simulink model "AreaCoverageTestHarness"  (R2016b)
settings: Solver=FixedStepDiscrete  StartTime=0.0  StopTime=1000  FixedStep=0.0001  RelTol=1e-3  EnableMultiTasking=on
StopFcn:
  | if strcmp(get_param('AreaCoverageTestHarness/Robot/DetailedMap', 'Commented'), 'off')
  | evalin('base', 'MapCoveragePercent(roomSim)');
  | disp('STOP');
  | end
values from neighbouring files (symbols this model uses):
  BLOCK_SIZE = double(CAL_BLOCK_SIZE)    [AreaCoverageCalib.m]    (also in room_V1.m = 20; room_V2.m = 20; room_V3.m = 20)
  CAL_B_NmPerW = 1.5    [MotorConfigurationSheet.m]
  CAL_CurrentScaling_A = 0.04    [MotorConfigurationSheet.m]
  CAL_flux_e = 0.3    [MotorConfigurationSheet.m]
  CAL_flux_t = 3.0    (= 3)    [MotorConfigurationSheet.m]
  CAL_Inertia_J = 0.03    [MotorConfigurationSheet.m]
  CAL_Re_ohm = 0.5    [MotorConfigurationSheet.m]
  CAL_SimInduct_H = 0.001    [MotorConfigurationSheet.m]
  EAST = 0    [AreaCoverageCalib.m]
  ERRVAL = 5    [AreaCoverageCalib.m]
  gearRatio = 12    [AreaCoverageCalib.m]
  halfWheel_mm = 60    [AreaCoverageCalib.m]
  initXSim = 38    [AreaCoverageCalib.m]
  initYSim = 50    [AreaCoverageCalib.m]
  NORTH = 270    [AreaCoverageCalib.m]
  NVM_AngleStoreFlg = true    [AreaCoverageCalib.m]
  NVM_EAST = uint16(CAL_EAST)    [AreaCoverageCalib.m]
  NVM_NORTH = uint16(CAL_NORTH)    [AreaCoverageCalib.m]
  NVM_SOUTH = uint16(CAL_SOUTH)    [AreaCoverageCalib.m]
  NVM_WEST = uint16(CAL_WEST)    [AreaCoverageCalib.m]
  ROB_LENG_m = 0.25    [AreaCoverageCalib.m]
  ROBO_LENG = 30    [realMapPlotter.m]    (also in roomDrawing.m)
  ROOM_SIDE_SIZE = double(CAL_ROOM_SIDE_SIZE)    [AreaCoverageCalib.m]    (also in room_V1.m = 20; room_V2.m = 20; room_V3.m = 20)
  SAMPLE_TIME = 0.001    [AreaCoverageCalib.m]
  SOUTH = 90    [AreaCoverageCalib.m]
  thetaMapBp = [0 : 0.1 : 360]    [AreaCoverageCalib.m]
  thetaMapTb = [thetaMapTb1, thetaMapTb2, thetaMapTb3, thetaMapTb4, thetaMapTb5]    [AreaCoverageCalib.m]
  WEST = 180    [AreaCoverageCalib.m]
undefined symbols (not defined in the file or in its folder): CAL_WheelDiameter_cm, DiscIntNeverNeededParam, ENU_BACKWARD, ENU_FORWARD
libraries: simulink x3, RobotControlLib x1
(part 1 of 3)
settings Model: Creator=oelkawok  LastModifiedBy=oelkawok
settings OptimizationCC: DefaultParameterBehavior=Inlined  UseDivisionForNetSlopeComputation=on  DefaultUnderspecifiedDataType=single  EfficientFloat2IntCast=on  LifeSpan=Inf
settings DebuggingCC: ConsistencyChecking=warning  SignalInfNanChecking=error  SignalRangeChecking=error  ReadBeforeWriteMsg=EnableAllAsError  WriteAfterWriteMsg=EnableAllAsError  WriteAfterReadMsg=EnableAllAsError  AlgebraicLoopMsg=error  ArtificialAlgebraicLoopMsg=error  SaveWithParameterizedLinksMsg=error  SignalResolutionControl=TryResolveAllWithWarning  BlockPriorityViolationMsg=error  MinStepSizeMsg=error  SolverPrmCheckMsg=error  InheritedTsInSrcMsg=error  SingleTaskRateTransMsg=error  TasksWithSamePriorityMsg=error  SigSpecEnsureSampleTimeMsg=error  CheckMatrixSingularityMsg=error  IntegerOverflowMsg=error  ParameterUnderflowMsg=error  UnderSpecifiedDataTypeMsg=warning  UnnecessaryDatatypeConvMsg=warning  VectorMatrixConversionMsg=error  SignalLabelMismatchMsg=error  UnconnectedLineMsg=error  SFcnCompatibilityMsg=warning  UniqueDataStoreMsg=error  BusObjectLabelMismatch=error  RootOutportRequireBusObject=error  AssertControl=DisableAll  ModelReferenceIOMsg=error  ModelReferenceVersionMismatchMessage=error  ModelReferenceIOMismatchMessage=error  UnknownTsInhSupMsg=error  ModelReferenceDataLoggingMessage=error  StateNameClashWarn=warning  StrictBusMsg=ErrorOnBusTreatedAsVector  NonBusSignalsTreatedAsBus=error  SFUnusedDataAndEventsDiag=error  SFInvalidInputDataAccessInChartInitDiag=error  SFTransitionOutsideNaturalParentDiag=error  SFUnreachableExecutionPathDiag=error  SFUndirectedBroadcastEventsDiag=error  SFTransitionActionBeforeConditionDiag=error  SFTemporalDelaySmallerThanSampleTimeDiag=error  SFSelfTransitionDiag=error  SFExecutionAtInitializationDiag=none  SFMachineParentedDataDiag=error
settings HardwareCC: ProdLongLongMode=on
settings RTWCC: SystemTargetFile=ert.tlc  TemplateMakefile=ert_default_tmf  Description=Embedded Coder  GenerateReport=on  IncludeHyperlinkInReport=on  LaunchReport=on  GenerateTraceInfo=on  GenerateTraceReport=on  GenerateTraceReportSl=on  GenerateTraceReportSf=on  GenerateTraceReportEml=on
settings CodeAppCC: ForceParamTrailComments=on  IgnoreCustomStorageClasses=off  OperatorAnnotations=on  SimulinkDataObjDesc=on  SFDataObjDesc=on  MATLABFcnDesc=on  InsertBlockDesc=on  MATLABSourceComments=on  ReqsInCode=on
settings ERTTargetCC: GenerateSampleERTMain=on  InlinedParameterPlacement=NonHierarchical  ERTCustomFileTemplate=example_file_process.tlc
settings ConfigComp: CovScope=ReferencedModels  CovIncludeTopModel=off  CovMetricSettings=dw  CovHtmlReporting=on  CovSaveCumulativeToWorkspaceVar=on  CovSaveSingleToWorkspaceVar=on  CovExternalEMLEnable=off

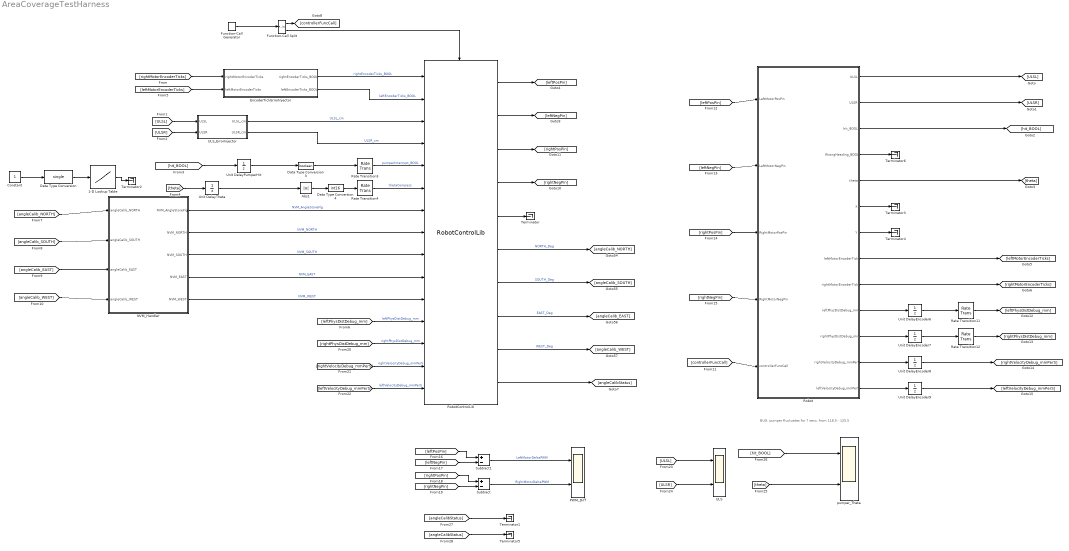
== system AreaCoverageTestHarness ==
  note: BUG: pumper fluctuates for 7 secs. from 118.5 - 125.5
  1-D Lookup Table : Lookup_n-D  NumberOfTableDimensions=1  BreakpointsForDimension1=thetaMapBp  Table=thetaMapTb  ExtrapMethod=Clip  InternalRulePriority=Speed  RndMeth=Simplest  InputSameDT=on
  Abs1 : Abs
  Constant : Constant
  Data Type Conversion : DataTypeConversion  OutDataTypeStr=single
  Data Type Conversion3 : DataTypeConversion  OutDataTypeStr=boolean
  Data Type Conversion4 : DataTypeConversion  OutDataTypeStr=int16
  EncoderTickErrorInjector : Subsystem
  Function-Call Generator : simulink/Ports & Subsystems/Function-Call Generator  sample_time=0.001  numberOfIterations=1
  Function-Call Split : FunctionCallSplit  IconShape=distinctive  NumOutputPorts=2  OutputPortLayout=default
  NVM_Handler : Subsystem
  PWM_Diff : Scope  NumInputPorts=2
  Rate Transition{3..4,11..12} (4 alike) : RateTransition
  Robot : Subsystem
  RobotControlLib : RobotControlLib/RobotControlLib  Description=Main Control Function
  Subtract : Sum  Inputs=+-  OutDataTypeStr=int16
  Subtract1 : Sum  Inputs=+-  OutDataTypeStr=int16
  Terminator{,1..6} (7 alike) : Terminator
  ULS : Scope  NumInputPorts=2
  ULS_ErrorInjector : Subsystem
  Unit DelayEncoder{6..9} (4 alike) : UnitDelay  SampleTime=-1
  Unit DelayPumperHit : UnitDelay  SampleTime=-1
      settings: AttributesFormatString=Init: %<InitialCondition>
  Unit DelayTheta : UnitDelay  InitialCondition=NORTH  SampleTime=-1
      settings: AttributesFormatString=%<InitialCondition>
  pumper_Theta : Scope  NumInputPorts=2
  wires:
  Data Type Conversion3/1 -> Rate Transition3/1
  Unit DelayPumperHit/1 -> Data Type Conversion3/1
  Abs1/1 -> Data Type Conversion4/1
  Robot/9(rightMotorEncoderTicks) -> [rightMotorEncoderTicks]
  Robot/1(ULSL) -> [ULSL]
  Robot/2(ULSR) -> [ULSR]
  Robot/3(hit_BOOL) -> [hit_BOOL]
  Robot/5(theta) -> [theta]
  Robot/8(leftMotorEncoderTicks) -> [leftMotorEncoderTicks]
  [hit_BOOL] -> Unit DelayPumperHit/1
  [theta] -> Unit DelayTheta/1
  RobotControlLib/10 -> [angleCalibStatus]
  RobotControlLib/6 -> [angleCalib_NORTH]  "NORTH_Deg"
  RobotControlLib/7 -> [angleCalib_SOUTH]  "SOUTH_Deg"
  RobotControlLib/8 -> [angleCalib_EAST]  "EAST_Deg"
  RobotControlLib/9 -> [angleCalib_WEST]  "WEST_Deg"
  Function-Call Generator/1 -> Function-Call Split/1
  [controllerFuncCall] -> Robot/5(controllerFuncCall)
  Function-Call Split/1 -> [controllerFuncCall]
  Function-Call Split/2 -> RobotControlLib/Trigger
  Rate Transition3/1 -> RobotControlLib/5  "pumperInterrupt_BOOL"
  Rate Transition4/1 -> RobotControlLib/6  "thetaCompass"
  Robot/10(leftPhysDistDebug_mm) -> Unit DelayEncoder6/1
  Robot/11(rightPhysDistDebug_mm) -> Unit DelayEncoder7/1
  Robot/12(rightVelocityDebug_mmPerS) -> Unit DelayEncoder8/1
  Robot/13(leftVelocityDebug_mmPerS) -> Unit DelayEncoder9/1
  Subtract/1 -> PWM_Diff/2  "RightMotorDeltaPWM"
  Subtract1/1 -> PWM_Diff/1  "LeftMotorDeltaPWM"
  RobotControlLib/1 -> [leftPosPin]
  RobotControlLib/2 -> [leftNegPin]
  RobotControlLib/3 -> [rightPosPin]
  RobotControlLib/4 -> [rightNegPin]
  [leftPosPin] -> Robot/1(LeftMotorPosPin)
  [leftNegPin] -> Robot/2(LeftMotorNegPin)
  [rightPosPin] -> Robot/3(RightMotorPosPin)
  [rightNegPin] -> Robot/4(RightMotorNegPin)
  [leftNegPin] -> Subtract1/2
  [leftPosPin] -> Subtract1/1
  [rightNegPin] -> Subtract/2
  [rightPosPin] -> Subtract/1
  [angleCalib_SOUTH] -> NVM_Handler/2(angleCalib_SOUTH)
  [angleCalib_NORTH] -> NVM_Handler/1(angleCalib_NORTH)
  [angleCalib_EAST] -> NVM_Handler/3(angleCalib_EAST)
  [angleCalib_WEST] -> NVM_Handler/4(angleCalib_WEST)
  Unit DelayEncoder6/1 -> Rate Transition11/1
  Rate Transition11/1 -> [leftPhysDistDebug_mm]
  [leftPhysDistDebug_mm] -> RobotControlLib/12  "leftPhysDistDebug_mm"
  Unit DelayEncoder7/1 -> Rate Transition12/1
  Rate Transition12/1 -> [rightPhysDistDebug_mm]
  [rightPhysDistDebug_mm] -> RobotControlLib/13  "rightPhysDistDebug_mm"
  Unit DelayEncoder8/1 -> [rightVelocityDebug_mmPerS]
  [rightVelocityDebug_mmPerS] -> RobotControlLib/14  "rightVelocityDebug_mmPerS"
  Unit DelayEncoder9/1 -> [leftVelocityDebug_mmPerS]
  [leftVelocityDebug_mmPerS] -> RobotControlLib/15  "leftVelocityDebug_mmPerS"
  NVM_Handler/5(NVM_WEST) -> RobotControlLib/11  "NVM_WEST"
  NVM_Handler/4(NVM_EAST) -> RobotControlLib/10  "NVM_EAST"
  NVM_Handler/3(NVM_SOUTH) -> RobotControlLib/9  "NVM_SOUTH"
  NVM_Handler/2(NVM_NORTH) -> RobotControlLib/8  "NVM_NORTH"
  NVM_Handler/1(NVM_AngleStoreFlg) -> RobotControlLib/7  "NVM_AngleStoreFlg"
  ULS_ErrorInjector/1(ULSL_cm) -> RobotControlLib/3  "ULSL_cm"
  ULS_ErrorInjector/2(ULSR_cm) -> RobotControlLib/4  "ULSR_cm"
  [ULSL] -> ULS_ErrorInjector/1(ULSL)
  [ULSR] -> ULS_ErrorInjector/2(ULSR)
  EncoderTickErrorInjector/1(rightEncoderTicks_BOOL) -> RobotControlLib/1  "rightEncoderTicks_BOOL"
  EncoderTickErrorInjector/2(leftEncoderTicks_BOOL) -> RobotControlLib/2  "leftEncoderTicks_BOOL"
  [leftMotorEncoderTicks] -> EncoderTickErrorInjector/2(leftMotorEncoderTicks)
  [rightMotorEncoderTicks] -> EncoderTickErrorInjector/1(rightMotorEncoderTicks)
  [ULSL] -> ULS/1
  [ULSR] -> ULS/2
  [theta] -> pumper_Theta/2
  [hit_BOOL] -> pumper_Theta/1
  Data Type Conversion4/1 -> Rate Transition4/1
  Unit DelayTheta/1 -> Abs1/1
  RobotControlLib/5 -> Terminator/1
  [angleCalibStatus] -> Terminator1/1
  Constant/1 -> Data Type Conversion/1
  1-D Lookup Table/1 -> Terminator2/1
  Robot/6(X) -> Terminator3/1
  Robot/7(Y) -> Terminator4/1
  [angleCalibStatus] -> Terminator5/1
  Robot/4(WrongHeading_BOOL) -> Terminator6/1
  Data Type Conversion/1 -> 1-D Lookup Table/1

== system AreaCoverageTestHarness/EncoderTickErrorInjector ==
  rightMotorEncoderTicks : Inport
  leftMotorEncoderTicks : Inport  Port=2
  Constant4 : Constant  Value=false
  Constant5 : Constant  Value=false
  Data Type Conversion1 : DataTypeConversion  OutDataTypeStr=boolean
  Data Type Conversion2 : DataTypeConversion  OutDataTypeStr=boolean
  Manual Switch2 : ManualSwitch
  Manual Switch3 : ManualSwitch
  Rate Transition : RateTransition
  Rate Transition5 : RateTransition
  Unit DelayEncoder : UnitDelay  SampleTime=-1
      settings: AttributesFormatString=init: %<InitialCondition>
  Unit DelayEncoder1 : UnitDelay  SampleTime=-1
      settings: AttributesFormatString=init: %<InitialCondition>
  rightEncoderTicks_BOOL : Outport
  leftEncoderTicks_BOOL : Outport  Port=2
  wires:
  Data Type Conversion2/1 -> Manual Switch3/1
  Unit DelayEncoder/1 -> Data Type Conversion2/1
  Constant5/1 -> Manual Switch3/2
  Manual Switch3/1 -> Rate Transition/1
  Rate Transition/1 -> rightEncoderTicks_BOOL/1
  Unit DelayEncoder1/1 -> Data Type Conversion1/1
  Constant4/1 -> Manual Switch2/2
  Manual Switch2/1 -> Rate Transition5/1
  Rate Transition5/1 -> leftEncoderTicks_BOOL/1
  Data Type Conversion1/1 -> Manual Switch2/1
  rightMotorEncoderTicks/1 -> Unit DelayEncoder/1
  leftMotorEncoderTicks/1 -> Unit DelayEncoder1/1

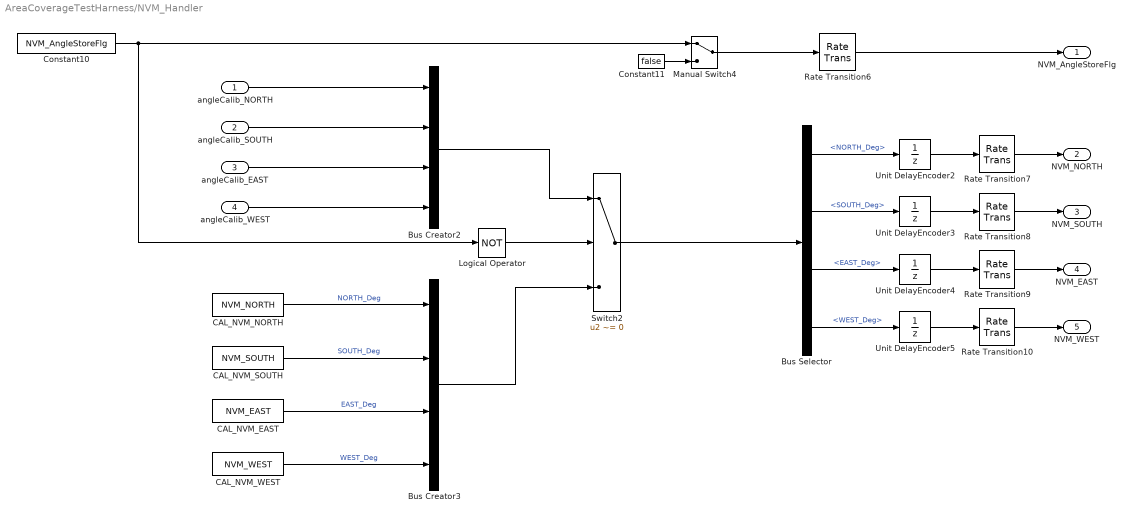
== system AreaCoverageTestHarness/NVM_Handler ==
  angleCalib_NORTH : Inport
  angleCalib_SOUTH : Inport  Port=2
  angleCalib_EAST : Inport  Port=3
  angleCalib_WEST : Inport  Port=4
  Bus Creator2 : BusCreator  Inputs=4
  Bus Creator3 : BusCreator  Inputs=4
  Bus Selector : BusSelector  OutputSignals=NORTH_Deg,SOUTH_Deg,EAST_Deg,WEST_Deg
  CAL_NVM_EAST : Constant  Value=NVM_EAST
  CAL_NVM_NORTH : Constant  Value=NVM_NORTH
  CAL_NVM_SOUTH : Constant  Value=NVM_SOUTH
  CAL_NVM_WEST : Constant  Value=NVM_WEST
  Constant10 : Constant  Value=NVM_AngleStoreFlg
  Constant11 : Constant  Value=false
  Logical Operator : Logic  Operator=NOT  IconShape=distinctive  AllPortsSameDT=off  OutDataTypeStr=boolean
  Manual Switch4 : ManualSwitch
  Rate Transition{6..10} (5 alike) : RateTransition
  Switch2 : Switch  Criteria=u2 ~= 0
  Unit DelayEncoder{2..5} (4 alike) : UnitDelay  SampleTime=-1
  NVM_AngleStoreFlg : Outport
  NVM_NORTH : Outport  Port=2
  NVM_SOUTH : Outport  Port=3
  NVM_EAST : Outport  Port=4
  NVM_WEST : Outport  Port=5
  wires:
  Constant10/1 -> Logical Operator/1, Manual Switch4/1
  Bus Creator2/1 -> Switch2/1
  Bus Creator3/1 -> Switch2/3
  Bus Selector/3 -> Unit DelayEncoder4/1  "<EAST_Deg>"
  Switch2/1 -> Bus Selector/1
  Bus Selector/4 -> Unit DelayEncoder5/1  "<WEST_Deg>"
  CAL_NVM_NORTH/1 -> Bus Creator3/1  "NORTH_Deg"
  CAL_NVM_EAST/1 -> Bus Creator3/3  "EAST_Deg"
  CAL_NVM_WEST/1 -> Bus Creator3/4  "WEST_Deg"
  Bus Selector/1 -> Unit DelayEncoder2/1  "<NORTH_Deg>"
  CAL_NVM_SOUTH/1 -> Bus Creator3/2  "SOUTH_Deg"
  Bus Selector/2 -> Unit DelayEncoder3/1  "<SOUTH_Deg>"
  Logical Operator/1 -> Switch2/2
  angleCalib_NORTH/1 -> Bus Creator2/1
  angleCalib_SOUTH/1 -> Bus Creator2/2
  angleCalib_WEST/1 -> Bus Creator2/4
  angleCalib_EAST/1 -> Bus Creator2/3
  Rate Transition10/1 -> NVM_WEST/1
  Rate Transition7/1 -> NVM_NORTH/1
  Rate Transition8/1 -> NVM_SOUTH/1
  Rate Transition9/1 -> NVM_EAST/1
  Manual Switch4/1 -> Rate Transition6/1
  Constant11/1 -> Manual Switch4/2
  Rate Transition6/1 -> NVM_AngleStoreFlg/1
  Unit DelayEncoder2/1 -> Rate Transition7/1
  Unit DelayEncoder3/1 -> Rate Transition8/1
  Unit DelayEncoder4/1 -> Rate Transition9/1
  Unit DelayEncoder5/1 -> Rate Transition10/1

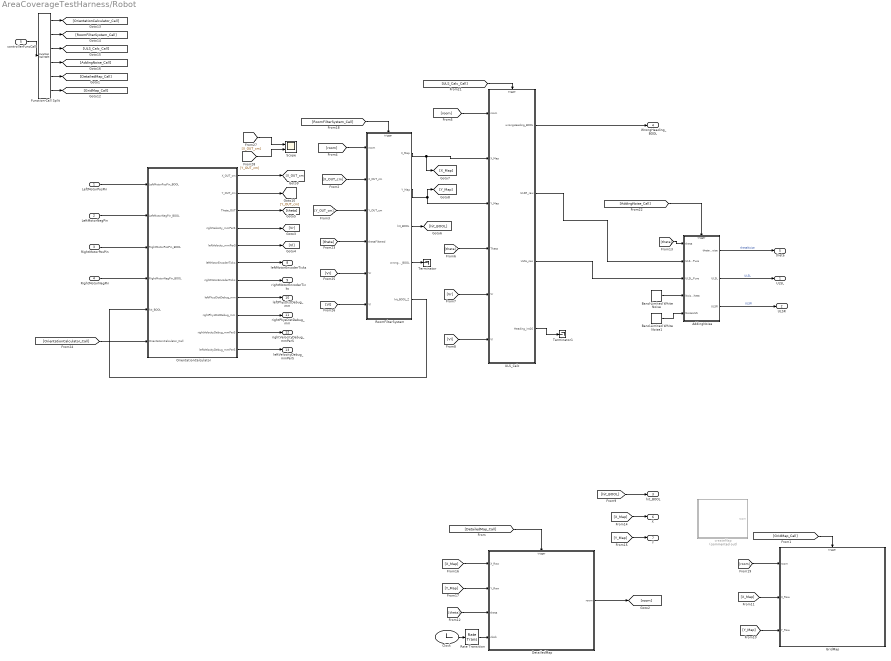
== system AreaCoverageTestHarness/Robot ==
  LeftMotorPosPin : Inport
  LeftMotorNegPin : Inport  Port=2
  RightMotorPosPin : Inport  Port=3
  RightMotorNegPin : Inport  Port=4
  controllerFuncCall : Inport  Port=5
  AddingNoise : Subsystem
  Band-Limited White Noise : simulink/Sources/Band-Limited White Noise  Cov=[0.001]  Ts=0.001  seed=[23]
  Band-Limited White Noise1 : simulink/Sources/Band-Limited White Noise  Cov=[0.001]  Ts=0.001  seed=[23]
  Clock : Clock
      settings: Decimation=100
  DetailedMap : Subsystem
  Function-Call Split : FunctionCallSplit  IconShape=distinctive  NumOutputPorts=6  OutputPortLayout=default
  GridMap : Subsystem
  OrientationCalculator : Subsystem
  Rate Transition : RateTransition
  RoomFilterSystem : Subsystem
  Scope : Scope  NumInputPorts=2
  Terminator : Terminator
  Terminator1 : Terminator
  ULS_Calc : Subsystem
  createMap : Subsystem  Commented=on
  ULSL : Outport
  ULSR : Outport  Port=2
  hit_BOOL : Outport  Port=3
  WrongHeading_BOOL : Outport  Port=4
  theta : Outport  Port=5
  X : Outport  Port=6
  Y : Outport  Port=7
  leftMotorEncoderTicks : Outport  Port=8
  rightMotorEncoderTicks : Outport  Port=9
  leftPhysDistDebug_mm : Outport  Port=10
  rightPhysDistDebug_mm : Outport  Port=11
  rightVelocityDebug_mmPerS : Outport  Port=12
  leftVelocityDebug_mmPerS : Outport  Port=13
  wires:
  RightMotorNegPin/1 -> OrientationCalculator/4(RightMotorNegPin_BOOL)
  RightMotorPosPin/1 -> OrientationCalculator/3(RightMotorPosPin_BOOL)
  OrientationCalculator/3(Theta_OUT) -> [theta]
  OrientationCalculator/4(rightVelocity_mmPerS) -> [Vr]
  RoomFilterSystem/3(hit_BOOL) -> [hit_BOOL]
  RoomFilterSystem/5(hit_BOOL_Z) -> OrientationCalculator/5(hit_BOOL)
  [room] -> RoomFilterSystem/1(room)
  [room] -> ULS_Calc/1(room)
  [theta] -> ULS_Calc/4(Theta)
  [Vr] -> ULS_Calc/5(Vr)
  [Vl] -> ULS_Calc/6(Vl)
  [hit_BOOL] -> hit_BOOL/1
  ULS_Calc/1(wrongHeading_BOOL) -> WrongHeading_BOOL/1
  RoomFilterSystem/2(Y_Map) -> ULS_Calc/3(Y_Map), [Y_Map]
  RoomFilterSystem/1(X_Map) -> [X_Map], ULS_Calc/2(X_Map)
  [Y_Map] -> Y/1
  [X_Map] -> X/1
  OrientationCalculator/1(X_OUT_cm) -> [X_OUT_cm]
  OrientationCalculator/2(Y_OUT_cm) -> [Y_OUT_cm]
  [X_Map] -> DetailedMap/1(X_Raw)
  [Y_Map] -> DetailedMap/2(Y_Raw)
  [theta] -> DetailedMap/3(theta)
  [X_Map] -> GridMap/2(X_Raw)
  [Y_Map] -> GridMap/3(Y_Raw)
  [room] -> GridMap/1(room)
  DetailedMap/1(room) -> [room]
  AddingNoise/2(ULSL) -> ULSL/1  "ULSL"
  AddingNoise/3(ULSR) -> ULSR/1  "ULSR"
  OrientationCalculator/6(leftMotorEncoderTicks) -> leftMotorEncoderTicks/1
  OrientationCalculator/7(rightMotorEncoderTicks) -> rightMotorEncoderTicks/1
  RoomFilterSystem/4(wrongHeading_BOOL) -> Terminator/1
  AddingNoise/1(thetaNoise) -> theta/1  "thetaNoise"
  [theta] -> AddingNoise/1(theta)
  ULS_Calc/3(ULSL_raw) -> AddingNoise/3(ULSL_Pure)
  [RoomFilterSystem_Call] -> RoomFilterSystem/Trigger
  [ULS_Calc_Call] -> ULS_Calc/Trigger
  [OrientationCalculator_Call] -> OrientationCalculator/6(OrientationCalculator_Call)
  controllerFuncCall/1 -> Function-Call Split/1
  ULS_Calc/2(ULSR_raw) -> AddingNoise/2(ULSR_Pure)
  [AddingNoise_Call] -> AddingNoise/Trigger
  Function-Call Split/4 -> [AddingNoise_Call]
  Function-Call Split/3 -> [ULS_Calc_Call]
  Function-Call Split/2 -> [RoomFilterSystem_Call]
  Function-Call Split/1 -> [OrientationCalculator_Call]
  Band-Limited White Noise1/1 -> AddingNoise/5(NoiseULS)
  Band-Limited White Noise/1 -> AddingNoise/4(NoiseTheta)
  OrientationCalculator/8(leftPhysDistDebug_mm) -> leftPhysDistDebug_mm/1
  OrientationCalculator/9(rightPhysDistDebug_mm) -> rightPhysDistDebug_mm/1
  OrientationCalculator/11(leftVelocityDebug_mmPerS) -> leftVelocityDebug_mmPerS/1
  OrientationCalculator/10(rightVelocityDebug_mmPerS) -> rightVelocityDebug_mmPerS/1
  LeftMotorPosPin/1 -> OrientationCalculator/1(LeftMotorPosPin_BOOL)
  LeftMotorNegPin/1 -> OrientationCalculator/2(LeftMotorNegPin_BOOL)
  Function-Call Split/5 -> [DetailedMap_Call]
  Function-Call Split/6 -> [GridMap_Call]
  [DetailedMap_Call] -> DetailedMap/Trigger
  [GridMap_Call] -> GridMap/Trigger
  Clock/1 -> Rate Transition/1
  Rate Transition/1 -> DetailedMap/4(clock)
  [X_OUT_cm] -> RoomFilterSystem/2(X_OUT_cm)
  [Y_OUT_cm] -> RoomFilterSystem/3(Y_OUT_cm)
  [theta] -> RoomFilterSystem/4(thetaFiltered)
  [Vr] -> RoomFilterSystem/5(Vr)
  OrientationCalculator/5(leftVelocity_mmPerS) -> [Vl]
  [Vl] -> RoomFilterSystem/6(Vl)
  [X_OUT_cm] -> Scope/1
  [Y_OUT_cm] -> Scope/2
  ULS_Calc/4(Heading_int16) -> Terminator1/1

== system AreaCoverageTestHarness/ULS_ErrorInjector ==
  ULSL : Inport
  ULSR : Inport  Port=2
  Abs2 : Abs
  Abs3 : Abs
  Constant : Constant  Value=0  OutDataTypeStr=uint16
  Constant2 : Constant  Value=0  OutDataTypeStr=uint16
  Data Type Conversion : DataTypeConversion  OutDataTypeStr=uint16
  Data Type Conversion1 : DataTypeConversion  OutDataTypeStr=uint16
  Manual Switch : ManualSwitch
  Manual Switch1 : ManualSwitch
  Rate Transition1 : RateTransition
  Rate Transition2 : RateTransition
  Unit DelayULSL : UnitDelay  InitialCondition=1  SampleTime=-1
  Unit DelayULSR : UnitDelay  InitialCondition=1  SampleTime=-1
  ULSL_cm : Outport
  ULSR_cm : Outport  Port=2
  wires:
  Manual Switch/1 -> Rate Transition1/1
  Abs3/1 -> Data Type Conversion1/1
  Abs2/1 -> Data Type Conversion/1
  Unit DelayULSL/1 -> Abs3/1
  Data Type Conversion/1 -> Manual Switch/1
  Data Type Conversion1/1 -> Manual Switch1/1
  Constant/1 -> Manual Switch/2
  Constant2/1 -> Manual Switch1/2
  Manual Switch1/1 -> Rate Transition2/1
  Unit DelayULSR/1 -> Abs2/1
  Rate Transition1/1 -> ULSL_cm/1
  Rate Transition2/1 -> ULSR_cm/1
  ULSR/1 -> Unit DelayULSL/1
  ULSL/1 -> Unit DelayULSR/1

== system AreaCoverageTestHarness/Robot/AddingNoise ==
  theta : Inport
  ULSR_Pure : Inport  Port=2
  ULSL_Pure : Inport  Port=3
  NoiseTheta : Inport  Port=4
  NoiseULS : Inport  Port=5
  function : TriggerPort  TriggerType=function-call  VariantControl=Variant
  Sum : Sum  Inputs=|++
  Sum1 : Sum  Inputs=|++
  Sum2 : Sum  Inputs=++|
  thetaNoise : Outport
  ULSL : Outport  Port=2
      settings: AttributesFormatString=%<OutputWhenDisabled>
  ULSR : Outport  Port=3
      settings: AttributesFormatString=%<OutputWhenDisabled>
  wires:
  NoiseTheta/1 -> Sum/2
  Sum/1 -> thetaNoise/1
  theta/1 -> Sum/1  "theta"
  ULSR_Pure/1 -> Sum1/1
  ULSL_Pure/1 -> Sum2/2
  NoiseULS/1 -> Sum1/2, Sum2/1
  Sum1/1 -> ULSR/1
  Sum2/1 -> ULSL/1

== system AreaCoverageTestHarness/Robot/DetailedMap ==
  X_Raw : Inport
  Y_Raw : Inport  Port=2
  theta : Inport  Port=3
  clock : Inport  Port=4
  function : TriggerPort  TriggerType=function-call  VariantControl=Variant
  MATLAB Function : MATLAB Function  TreatAsAtomicUnit=on
  createMap : Subsystem  Variant=on  OverrideUsingVariant=Variant
  room : Outport
  wires:
  theta/1 -> MATLAB Function/4(Theta)
  createMap/1(room) -> room/1, MATLAB Function/1(room)
  X_Raw/1 -> MATLAB Function/2(X)
  Y_Raw/1 -> MATLAB Function/3(Y)
  clock/1 -> MATLAB Function/5(clock)

== system AreaCoverageTestHarness/Robot/GridMap ==
  room : Inport
  X_Raw : Inport  Port=2
  Y_Raw : Inport  Port=3
  function : TriggerPort  TriggerType=function-call  VariantControl=Variant
  MATLAB Function : MATLAB Function  TreatAsAtomicUnit=on
  wires:
  Y_Raw/1 -> MATLAB Function/3(Y)
  X_Raw/1 -> MATLAB Function/2(X)
  room/1 -> MATLAB Function/1(room)

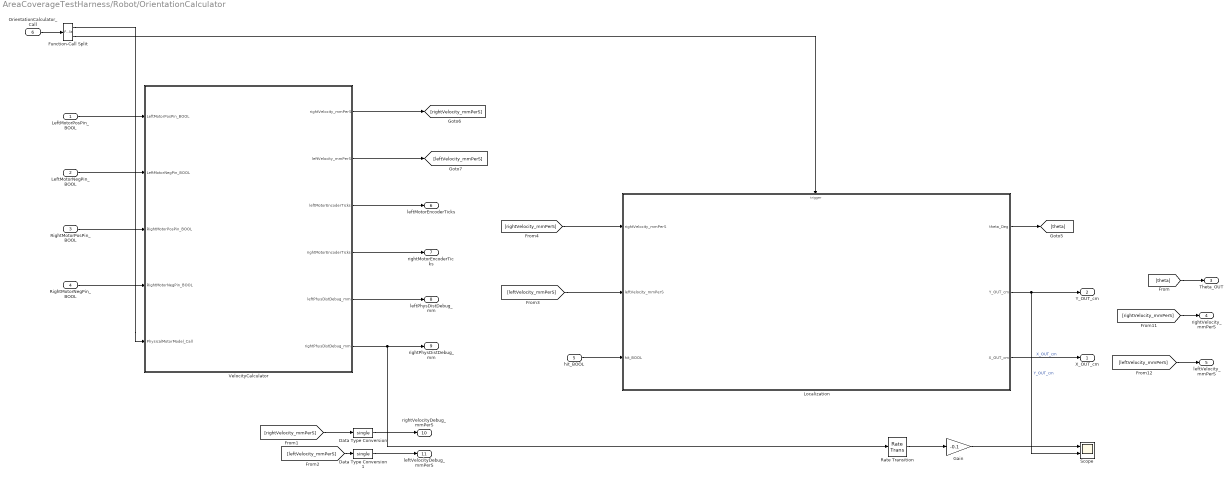
== system AreaCoverageTestHarness/Robot/OrientationCalculator ==
  LeftMotorPosPin_BOOL : Inport
  LeftMotorNegPin_BOOL : Inport  Port=2
  RightMotorPosPin_BOOL : Inport  Port=3
  RightMotorNegPin_BOOL : Inport  Port=4
  hit_BOOL : Inport  Port=5
  OrientationCalculator_Call : Inport  Port=6
  Data Type Conversion : DataTypeConversion  OutDataTypeStr=single
  Data Type Conversion1 : DataTypeConversion  OutDataTypeStr=single
  Function-Call Split : FunctionCallSplit  IconShape=distinctive  NumOutputPorts=2
  Gain : Gain  Gain=-0.1
  Localization : Subsystem
  Rate Transition : RateTransition
  Scope : Scope  NumInputPorts=2
  VelocityCalculator : Subsystem
  X_OUT_cm : Outport
  Y_OUT_cm : Outport  Port=2
  Theta_OUT : Outport  Port=3
  rightVelocity_mmPerS : Outport  Port=4
  leftVelocity_mmPerS : Outport  Port=5
  leftMotorEncoderTicks : Outport  Port=6
  rightMotorEncoderTicks : Outport  Port=7
  leftPhysDistDebug_mm : Outport  Port=8
  rightPhysDistDebug_mm : Outport  Port=9
  rightVelocityDebug_mmPerS : Outport  Port=10
  leftVelocityDebug_mmPerS : Outport  Port=11
  wires:
  [leftVelocity_mmPerS] -> leftVelocity_mmPerS/1
  [rightVelocity_mmPerS] -> rightVelocity_mmPerS/1
  Localization/1(theta_Deg) -> [theta]
  [theta] -> Theta_OUT/1
  VelocityCalculator/3(leftMotorEncoderTicks) -> leftMotorEncoderTicks/1
  VelocityCalculator/4(rightMotorEncoderTicks) -> rightMotorEncoderTicks/1
  Localization/2(Y_OUT_cm) -> Scope/2, Y_OUT_cm/1  "Y_OUT_cm"
  Localization/3(X_OUT_cm) -> X_OUT_cm/1  "X_OUT_cm"
  hit_BOOL/1 -> Localization/3(hit_BOOL)
  LeftMotorPosPin_BOOL/1 -> VelocityCalculator/1(LeftMotorPosPin_BOOL)
  RightMotorNegPin_BOOL/1 -> VelocityCalculator/4(RightMotorNegPin_BOOL)
  RightMotorPosPin_BOOL/1 -> VelocityCalculator/3(RightMotorPosPin_BOOL)
  LeftMotorNegPin_BOOL/1 -> VelocityCalculator/2(LeftMotorNegPin_BOOL)
  VelocityCalculator/1(rightVelocity_mmPerS) -> [rightVelocity_mmPerS]
  VelocityCalculator/2(leftVelocity_mmPerS) -> [leftVelocity_mmPerS]
  OrientationCalculator_Call/1 -> Function-Call Split/1
  Function-Call Split/2 -> Localization/Trigger
  Function-Call Split/1 -> VelocityCalculator/5(PhysicalMotorModel_Call)
  VelocityCalculator/5(leftPhysDistDebug_mm) -> leftPhysDistDebug_mm/1
  VelocityCalculator/6(rightPhysDistDebug_mm) -> Rate Transition/1, rightPhysDistDebug_mm/1
  [rightVelocity_mmPerS] -> Data Type Conversion/1
  [leftVelocity_mmPerS] -> Data Type Conversion1/1
  Data Type Conversion/1 -> rightVelocityDebug_mmPerS/1
  Data Type Conversion1/1 -> leftVelocityDebug_mmPerS/1
  Rate Transition/1 -> Gain/1
  Gain/1 -> Scope/1
  [rightVelocity_mmPerS] -> Localization/1(rightVelocity_mmPerS)
  [leftVelocity_mmPerS] -> Localization/2(leftVelocity_mmPerS)

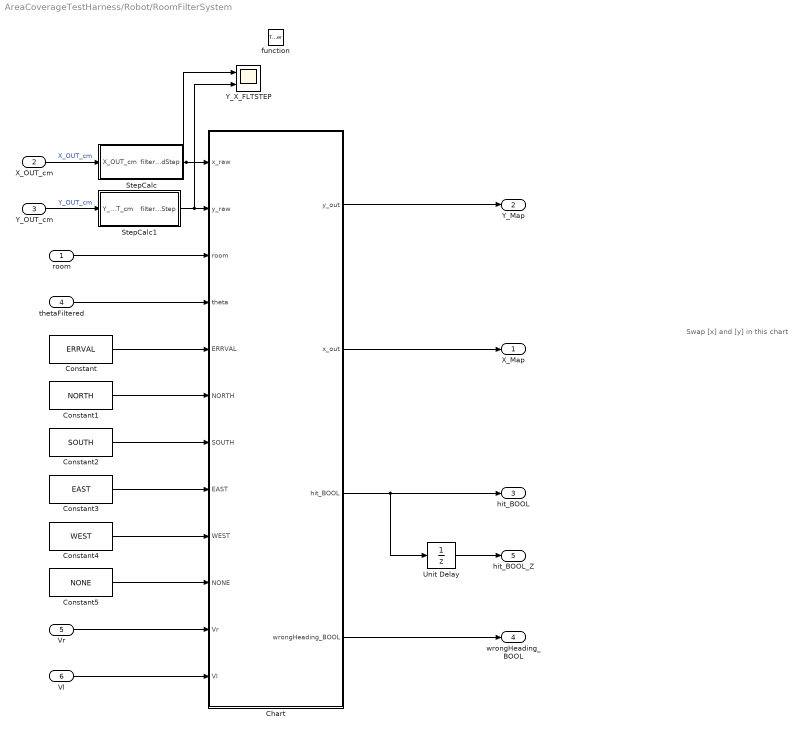
== system AreaCoverageTestHarness/Robot/RoomFilterSystem ==
  note: Swap [x] and [y] in this chart
  room : Inport
  X_OUT_cm : Inport  Port=2
  Y_OUT_cm : Inport  Port=3
  thetaFiltered : Inport  Port=4
  Vr : Inport  Port=5
  Vl : Inport  Port=6
  function : TriggerPort  TriggerType=function-call  VariantControl=Variant
  Chart : Stateflow chart  TreatAsAtomicUnit=on
  Constant : Constant  Value=ERRVAL
  Constant1 : Constant  Value=NORTH
  Constant2 : Constant  Value=SOUTH
  Constant3 : Constant  Value=EAST
  Constant4 : Constant  Value=WEST
  Constant5 : Constant  Value=NONE
  StepCalc : Subsystem
  StepCalc1 : Subsystem
  Unit Delay : UnitDelay  SampleTime=-1
      settings: AttributesFormatString=%<InitialCondition>
  Y_X_FLTSTEP : Scope  NumInputPorts=2
  X_Map : Outport
  Y_Map : Outport  Port=2
  hit_BOOL : Outport  Port=3
  wrongHeading_BOOL : Outport  Port=4
  hit_BOOL_Z : Outport  Port=5
  wires:
  Y_OUT_cm/1 -> StepCalc1/1(Y_OUT_cm)  "Y_OUT_cm"
  room/1 -> Chart/3(room)
  Chart/1(y_out) -> Y_Map/1
  Chart/2(x_out) -> X_Map/1
  thetaFiltered/1 -> Chart/4(theta)
  Constant/1 -> Chart/5(ERRVAL)
  Constant1/1 -> Chart/6(NORTH)
  Constant2/1 -> Chart/7(SOUTH)
  Constant5/1 -> Chart/10(NONE)
  Constant4/1 -> Chart/9(WEST)
  Constant3/1 -> Chart/8(EAST)
  Vr/1 -> Chart/11(Vr)
  Vl/1 -> Chart/12(Vl)
  Chart/3(hit_BOOL) -> Unit Delay/1, hit_BOOL/1
  Chart/4(wrongHeading_BOOL) -> wrongHeading_BOOL/1
  StepCalc1/1(filteredStep) -> Y_X_FLTSTEP/2, Chart/2(y_raw)
  X_OUT_cm/1 -> StepCalc/1(X_OUT_cm)  "X_OUT_cm"
  StepCalc/1(filteredStep) -> Y_X_FLTSTEP/1, Chart/1(x_raw)
  Unit Delay/1 -> hit_BOOL_Z/1

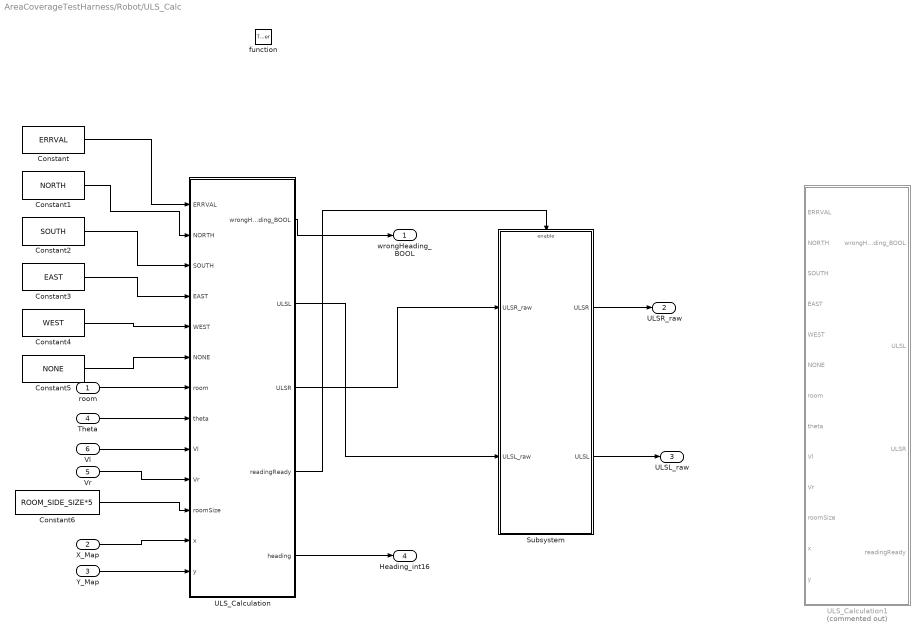
== system AreaCoverageTestHarness/Robot/ULS_Calc ==
  room : Inport
  X_Map : Inport  Port=2
  Y_Map : Inport  Port=3
  Theta : Inport  Port=4
  Vr : Inport  Port=5
  Vl : Inport  Port=6
  function : TriggerPort  TriggerType=function-call  VariantControl=Variant
  Constant : Constant  Value=ERRVAL
  Constant1 : Constant  Value=NORTH
  Constant2 : Constant  Value=SOUTH
  Constant3 : Constant  Value=EAST
  Constant4 : Constant  Value=WEST
  Constant5 : Constant  Value=NONE
  Constant6 : Constant  Value=ROOM_SIDE_SIZE*5
  Subsystem : Subsystem
  ULS_Calculation : Stateflow chart  TreatAsAtomicUnit=on
  ULS_Calculation1 : Stateflow chart  Commented=on  TreatAsAtomicUnit=on
  wrongHeading_BOOL : Outport
  ULSR_raw : Outport  Port=2
  ULSL_raw : Outport  Port=3
  Heading_int16 : Outport  Port=4
  wires:
  X_Map/1 -> ULS_Calculation/12(x)
  Y_Map/1 -> ULS_Calculation/13(y)
  Theta/1 -> ULS_Calculation/8(theta)
  Constant4/1 -> ULS_Calculation/5(WEST)
  Constant5/1 -> ULS_Calculation/6(NONE)
  Constant3/1 -> ULS_Calculation/4(EAST)
  Constant2/1 -> ULS_Calculation/3(SOUTH)
  Constant1/1 -> ULS_Calculation/2(NORTH)
  Constant/1 -> ULS_Calculation/1(ERRVAL)
  room/1 -> ULS_Calculation/7(room)
  Constant6/1 -> ULS_Calculation/11(roomSize)
  Vl/1 -> ULS_Calculation/9(Vl)
  Vr/1 -> ULS_Calculation/10(Vr)
  ULS_Calculation/4(readingReady) -> Subsystem/Enable
  ULS_Calculation/1(wrongHeading_BOOL) -> wrongHeading_BOOL/1
  ULS_Calculation/5(heading) -> Heading_int16/1
  Subsystem/1(ULSR) -> ULSR_raw/1
  Subsystem/2(ULSL) -> ULSL_raw/1
  ULS_Calculation/3(ULSR) -> Subsystem/1(ULSR_raw)
  ULS_Calculation/2(ULSL) -> Subsystem/2(ULSL_raw)

== system AreaCoverageTestHarness/Robot/createMap ==
  MATLAB Function : MATLAB Function  TreatAsAtomicUnit=on
  room : Outport
  wires:
  MATLAB Function/1(roomOut) -> room/1

== system AreaCoverageTestHarness/Robot/DetailedMap/createMap ==
  RoomV1 : Subsystem  VariantControl=Variant
  RoomV2 : Subsystem  VariantControl=Variant2
  RoomV3 : Subsystem  VariantControl=Variant3
  room : Outport

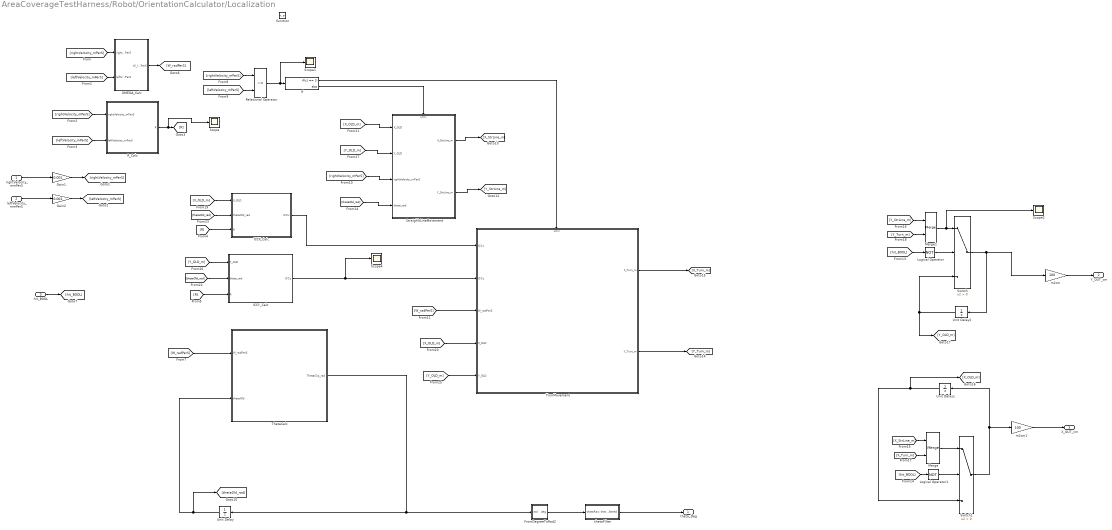
== system AreaCoverageTestHarness/Robot/OrientationCalculator/Localization ==
  rightVelocity_mmPerS : Inport
  leftVelocity_mmPerS : Inport  Port=2
  hit_BOOL : Inport  Port=3
  function : TriggerPort  TriggerType=function-call  VariantControl=Variant
  FromDegreeToRad2 : Subsystem
  Gain1 : Gain  Gain=0.001
  Gain2 : Gain  Gain=0.001
  ICCX_Calc : Subsystem
  ICCY_Calc : Subsystem
  If : If  IfExpression=u1 == 1
  Logical Operator : Logic  Operator=NOT  AllPortsSameDT=off  OutDataTypeStr=boolean
  Logical Operator1 : Logic  Operator=NOT  AllPortsSameDT=off  OutDataTypeStr=boolean
  Merge : Merge
  Merge1 : Merge
  OMEGA_Calc : Subsystem
  R_Calc : Subsystem
  Relational Operator : RelationalOperator  Operator=~=  OutDataTypeStr=boolean  RndMeth=Nearest
  Scope{,1..2,4} (4 alike) : Scope
  StraighltLineMovement : Subsystem  TreatAsAtomicUnit=on
  Switch : Switch  Criteria=u2 > Threshold
  Switch1 : Switch  Criteria=u2 > Threshold
  ThetaCalc : Subsystem
  TurnMovement : Subsystem
  Unit Delay : UnitDelay  InitialCondition=(NORTH*pi)/180  SampleTime=-1
      settings: AttributesFormatString=%<InitialCondition>
  Unit Delay1 : UnitDelay  InitialCondition=initXSim*0.01  SampleTime=-1
      settings: AttributesFormatString=%<InitialCondition>
  Unit Delay2 : UnitDelay  InitialCondition=initYSim*0.01  SampleTime=-1
      settings: AttributesFormatString=%<InitialCondition>
  m2cm : Gain  Gain=100
  m2cm1 : Gain  Gain=100
  thetaFilter : Subsystem
  theta_Deg : Outport
  Y_OUT_cm : Outport  Port=2
  X_OUT_cm : Outport  Port=3
  wires:
  [Y_OLD_m] -> TurnMovement/5(Y_OLD)
  [thetaOld_rad] -> ICCY_Calc/2(theta_rad)
  OMEGA_Calc/1(W_radPerS) -> [W_radPerS]
  ICCY_Calc/1(ICCy) -> Scope4/1, TurnMovement/2(ICCy)
  ICCX_Calc/1(ICCx) -> TurnMovement/1(ICCx)
  [R] -> ICCY_Calc/3(R)
  [R] -> ICCX_Calc/3(R)
  R_Calc/1(R) -> Scope/1, [R]
  [leftVelocity_mPerS] -> R_Calc/2(leftVelocity_mPerS)
  [rightVelocity_mPerS] -> R_Calc/1(rightVelocity_mPerS)
  [leftVelocity_mPerS] -> OMEGA_Calc/2(leftVelocity_mPerS)
  [rightVelocity_mPerS] -> OMEGA_Calc/1(rightVelocity_mPerS)
  If/2 -> StraighltLineMovement/Action
  If/1 -> TurnMovement/Action
  Relational Operator/1 -> Scope1/1, If/1
  [rightVelocity_mPerS] -> Relational Operator/1
  [leftVelocity_mPerS] -> Relational Operator/2
  [W_radPerS] -> TurnMovement/3(W_radPerS)
  [X_OLD_m] -> TurnMovement/4(X_OLD)
  [X_OLD_m] -> ICCX_Calc/1(X_OLD)
  [thetaOld_rad] -> ICCX_Calc/2(thetaOld_rad)
  [thetaOld_rad] -> StraighltLineMovement/4(theta_rad)
  TurnMovement/1(X_Turn_m) -> [X_Turn_m]
  StraighltLineMovement/1(X_StrLine_m) -> [X_StrLine_m]
  [Y_OLD_m] -> StraighltLineMovement/2(Y_OLD)
  [Y_OLD_m] -> ICCY_Calc/1(Y_OLD)
  [X_OLD_m] -> StraighltLineMovement/1(X_OLD)
  rightVelocity_mmPerS/1 -> Gain1/1
  leftVelocity_mmPerS/1 -> Gain2/1
  Unit Delay/1 -> [thetaOld_rad], ThetaCalc/2(thetaOld)
  ThetaCalc/1(ThetaClip_rad) -> FromDegreeToRad2/1(rad), Unit Delay/1
  [W_radPerS] -> ThetaCalc/1(W_radPerS)
  thetaFilter/1(thetaFiltered) -> theta_Deg/1
  Unit Delay1/1 -> Switch1/3, [X_OLD_m]
  [Y_StrLine_m] -> Merge1/1
  Merge1/1 -> Scope2/1, Switch/1
  [X_Turn_m] -> Merge/2
  [hit_BOOL] -> Logical Operator/1
  Logical Operator1/1 -> Switch1/2
  Switch1/1 -> m2cm1/1, Unit Delay1/1
  Unit Delay2/1 -> [Y_OLD_m], Switch/3
  Merge/1 -> Switch1/1
  [hit_BOOL] -> Logical Operator1/1
  [X_StrLine_m] -> Merge/1
  [Y_Turn_m] -> Merge1/2
  Logical Operator/1 -> Switch/2
  hit_BOOL/1 -> [hit_BOOL]
  StraighltLineMovement/2(Y_StrLine_m) -> [Y_StrLine_m]
  TurnMovement/2(Y_Turn_m) -> [Y_Turn_m]
  [rightVelocity_mPerS] -> StraighltLineMovement/3(rightVelocity_mPerS)
  Gain2/1 -> [leftVelocity_mPerS]
  Gain1/1 -> [rightVelocity_mPerS]
  FromDegreeToRad2/1(deg) -> thetaFilter/1(thetaRaw)
  m2cm/1 -> Y_OUT_cm/1
  m2cm1/1 -> X_OUT_cm/1
  Switch/1 -> m2cm/1, Unit Delay2/1

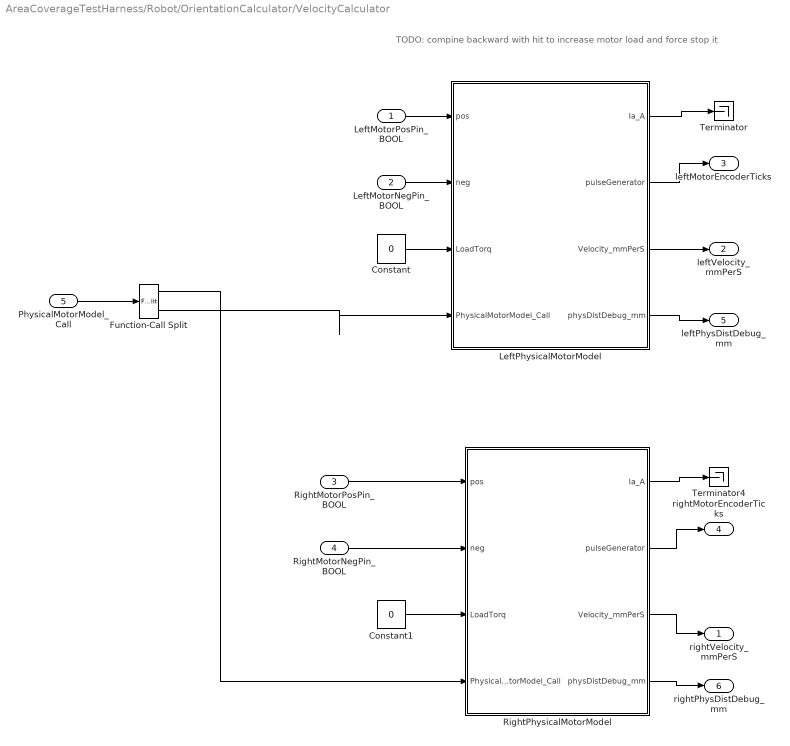
== system AreaCoverageTestHarness/Robot/OrientationCalculator/VelocityCalculator ==
  note: TODO: compine backward with hit to increase motor load and force stop it
  LeftMotorPosPin_BOOL : Inport
  LeftMotorNegPin_BOOL : Inport  Port=2
  RightMotorPosPin_BOOL : Inport  Port=3
  RightMotorNegPin_BOOL : Inport  Port=4
  PhysicalMotorModel_Call : Inport  Port=5
  Constant : Constant  Value=0
  Constant1 : Constant  Value=0
  Function-Call Split : FunctionCallSplit  IconShape=distinctive  NumOutputPorts=2
  LeftPhysicalMotorModel : Subsystem
  RightPhysicalMotorModel : Subsystem
  Terminator : Terminator
  Terminator4 : Terminator
  rightVelocity_mmPerS : Outport
  leftVelocity_mmPerS : Outport  Port=2
  leftMotorEncoderTicks : Outport  Port=3
  rightMotorEncoderTicks : Outport  Port=4
  leftPhysDistDebug_mm : Outport  Port=5
  rightPhysDistDebug_mm : Outport  Port=6
  wires:
  LeftMotorPosPin_BOOL/1 -> LeftPhysicalMotorModel/1(pos)
  LeftMotorNegPin_BOOL/1 -> LeftPhysicalMotorModel/2(neg)
  Constant/1 -> LeftPhysicalMotorModel/3(LoadTorq)
  LeftPhysicalMotorModel/1(Ia_A) -> Terminator/1
  LeftPhysicalMotorModel/3(Velocity_mmPerS) -> leftVelocity_mmPerS/1
  LeftPhysicalMotorModel/2(pulseGenerator) -> leftMotorEncoderTicks/1
  RightMotorNegPin_BOOL/1 -> RightPhysicalMotorModel/2(neg)
  Constant1/1 -> RightPhysicalMotorModel/3(LoadTorq)
  RightPhysicalMotorModel/1(Ia_A) -> Terminator4/1
  RightPhysicalMotorModel/2(pulseGenerator) -> rightMotorEncoderTicks/1
  RightMotorPosPin_BOOL/1 -> RightPhysicalMotorModel/1(pos)
  RightPhysicalMotorModel/3(Velocity_mmPerS) -> rightVelocity_mmPerS/1
  LeftPhysicalMotorModel/4(physDistDebug_mm) -> leftPhysDistDebug_mm/1
  PhysicalMotorModel_Call/1 -> Function-Call Split/1
  Function-Call Split/2 -> LeftPhysicalMotorModel/4(PhysicalMotorModel_Call)
  Function-Call Split/1 -> RightPhysicalMotorModel/4(PhysicalMotorModel_Call)
  RightPhysicalMotorModel/4(physDistDebug_mm) -> rightPhysDistDebug_mm/1

== system AreaCoverageTestHarness/Robot/RoomFilterSystem/StepCalc ==
  X_OUT_cm : Inport
  Chart : Stateflow chart  TreatAsAtomicUnit=on
  Data Type Conversion : DataTypeConversion  OutDataTypeStr=int32
  STEP_SIZE : Constant  Value=BLOCK_SIZE/4  OutDataTypeStr=int8
  Unit Delay : UnitDelay  SampleTime=-1
      settings: AttributesFormatString=%<InitialCondition>
  filteredStep : Outport
  wires:
  X_OUT_cm/1 -> Data Type Conversion/1
  Unit Delay/1 -> Chart/2(oldPos)
  Chart/1(step) -> filteredStep/1
  Data Type Conversion/1 -> Chart/1(pos), Unit Delay/1
  STEP_SIZE/1 -> Chart/3(STEP_SIZE)

== system AreaCoverageTestHarness/Robot/RoomFilterSystem/StepCalc1 ==
  Y_OUT_cm : Inport
  Chart : Stateflow chart  TreatAsAtomicUnit=on
  Data Type Conversion : DataTypeConversion  OutDataTypeStr=int32
  STEP_SIZE : Constant  Value=BLOCK_SIZE/4  OutDataTypeStr=int8
  Unit Delay : UnitDelay  SampleTime=-1
      settings: AttributesFormatString=%<InitialCondition>
  filteredStep : Outport
  wires:
  STEP_SIZE/1 -> Chart/3(STEP_SIZE)
  Data Type Conversion/1 -> Unit Delay/1, Chart/1(pos)
  Chart/1(step) -> filteredStep/1
  Unit Delay/1 -> Chart/2(oldPos)
  Y_OUT_cm/1 -> Data Type Conversion/1

== system AreaCoverageTestHarness/Robot/ULS_Calc/Subsystem ==
  ULSR_raw : Inport
  ULSL_raw : Inport  Port=2
  Enable : EnablePort
      settings: AttributesFormatString=%<StatesWhenEnabling>
  Constant : Constant  Value=ROBO_LENG
  Constant1 : Constant  Value=ROBO_LENG
  Gain : Gain  Gain=BLOCK_SIZE/4
  Gain1 : Gain  Gain=BLOCK_SIZE/4
  Gain2 : Gain  Gain=0.5
  Gain3 : Gain  Gain=0.5
  Subtract : Sum  Inputs=+-
  Subtract1 : Sum  Inputs=+-
  ULSR : Outport
      settings: AttributesFormatString=%<OutputWhenDisabled>
  ULSL : Outport  Port=2
      settings: AttributesFormatString=%<OutputWhenDisabled>
  wires:
  ULSL_raw/1 -> Gain1/1
  ULSR_raw/1 -> Gain/1
  Gain1/1 -> Subtract1/1
  Gain/1 -> Subtract/1
  Constant/1 -> Gain2/1
  Gain2/1 -> Subtract/2
  Constant1/1 -> Gain3/1
  Gain3/1 -> Subtract1/2
  Subtract/1 -> ULSR/1
  Subtract1/1 -> ULSL/1

== system AreaCoverageTestHarness/Robot/DetailedMap/createMap/RoomV1 ==
  Room_V1 : MATLAB Function  TreatAsAtomicUnit=on
  room : Outport
  wires:
  Room_V1/1(roomOut) -> room/1

== system AreaCoverageTestHarness/Robot/DetailedMap/createMap/RoomV2 ==
  Room_V2 : MATLAB Function  TreatAsAtomicUnit=on
  room : Outport
  wires:
  Room_V2/1(roomOut) -> room/1

== system AreaCoverageTestHarness/Robot/DetailedMap/createMap/RoomV3 ==
  Room_V3 : MATLAB Function  TreatAsAtomicUnit=on
  room : Outport
  wires:
  Room_V3/1(roomOut) -> room/1

== system AreaCoverageTestHarness/Robot/OrientationCalculator/Localization/FromDegreeToRad2 ==
  rad : Inport
  Constant1 : Constant  Value=pi
  Constant2 : Constant  Value=180
  Divide : Product  Inputs=*/
  Product : Product
  deg : Outport
  wires:
  Divide/1 -> Product/1
  rad/1 -> Product/2
  Product/1 -> deg/1
  Constant2/1 -> Divide/1
  Constant1/1 -> Divide/2

== system AreaCoverageTestHarness/Robot/OrientationCalculator/Localization/ICCX_Calc ==
  X_OLD : Inport
  thetaOld_rad : Inport  Port=2
  R : Inport  Port=3
  Product : Product
  Subtract : Sum  Inputs=+-
  Trigonometric Function1 : Trigonometry
  ICCx : Outport
  wires:
  Product/1 -> Subtract/2
  X_OLD/1 -> Subtract/1
  Subtract/1 -> ICCx/1
  Trigonometric Function1/1 -> Product/2
  R/1 -> Product/1
  thetaOld_rad/1 -> Trigonometric Function1/1

== system AreaCoverageTestHarness/Robot/OrientationCalculator/Localization/ICCY_Calc ==
  Y_OLD : Inport
  theta_rad : Inport  Port=2
  R : Inport  Port=3
  Product : Product
  Subtract : Sum
  Trigonometric Function1 : Trigonometry  Operator=cos
  ICCy : Outport
  wires:
  Y_OLD/1 -> Subtract/1
  Trigonometric Function1/1 -> Product/2
  Subtract/1 -> ICCy/1
  Product/1 -> Subtract/2
  R/1 -> Product/1
  theta_rad/1 -> Trigonometric Function1/1

== system AreaCoverageTestHarness/Robot/OrientationCalculator/Localization/OMEGA_Calc ==
  rightVelocity_mPerS : Inport
  leftVelocity_mPerS : Inport  Port=2
  Add : Sum  Inputs=+-
  Divide1 : Product  Inputs=*/
  ROB_LENG_m : Constant  Value=ROB_LENG_m
  W_radPerS : Outport
  wires:
  ROB_LENG_m/1 -> Divide1/2
  Divide1/1 -> W_radPerS/1  "w"
  Add/1 -> Divide1/1
  leftVelocity_mPerS/1 -> Add/1
  rightVelocity_mPerS/1 -> Add/2

== system AreaCoverageTestHarness/Robot/OrientationCalculator/Localization/R_Calc ==
  rightVelocity_mPerS : Inport
  leftVelocity_mPerS : Inport  Port=2
  If : If  NumInputs=2  IfExpression=u1 ~= u2  ShowElse=off
  If Action Subsystem1 : Subsystem  TreatAsAtomicUnit=on
  R : Outport
  wires:
  If/1 -> If Action Subsystem1/Action
  If Action Subsystem1/1(R) -> R/1
  rightVelocity_mPerS/1 -> If Action Subsystem1/1(rightVelocity_mPerS), If/1
  leftVelocity_mPerS/1 -> If/2, If Action Subsystem1/2(leftVelocity_mPerS)

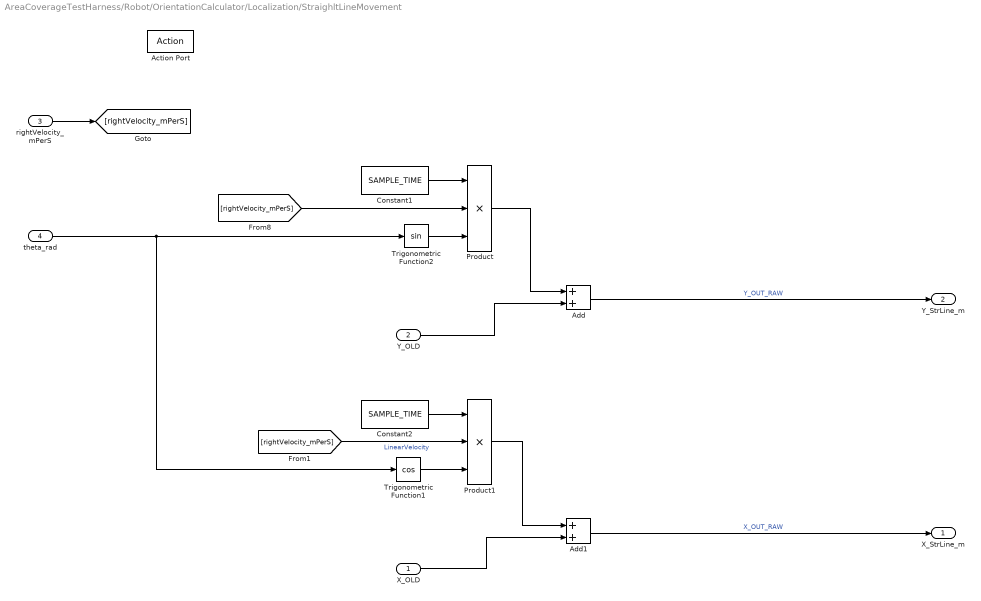
== system AreaCoverageTestHarness/Robot/OrientationCalculator/Localization/StraighltLineMovement ==
  X_OLD : Inport
  Y_OLD : Inport  Port=2
  rightVelocity_mPerS : Inport  Port=3
  theta_rad : Inport  Port=4
  Action Port : ActionPort  ActionType=else
      settings: AttributesFormatString=%<InitializeStates>
  Add : Sum
  Add1 : Sum
  Constant1 : Constant  Value=SAMPLE_TIME  SampleTime=-1
  Constant2 : Constant  Value=SAMPLE_TIME  SampleTime=-1
  Product : Product  Inputs=3
  Product1 : Product  Inputs=3
  Trigonometric Function1 : Trigonometry  Operator=cos
  Trigonometric Function2 : Trigonometry
  X_StrLine_m : Outport  InitialOutput=initXSim
      settings: AttributesFormatString=|
      | %<InitialOutput>
      | %<OutputWhenDisabled>
  Y_StrLine_m : Outport  Port=2  InitialOutput=initYSim
      settings: AttributesFormatString=|
      | %<InitialOutput>
      | %<OutputWhenDisabled>
  wires:
  rightVelocity_mPerS/1 -> [rightVelocity_mPerS]
  Constant1/1 -> Product/1
  Y_OLD/1 -> Add/2
  Product/1 -> Add/1
  Add/1 -> Y_StrLine_m/1  "Y_OUT_RAW"
  Constant2/1 -> Product1/1
  X_OLD/1 -> Add1/2
  Product1/1 -> Add1/1
  Add1/1 -> X_StrLine_m/1  "X_OUT_RAW"
  [rightVelocity_mPerS] -> Product1/2  "LinearVelocity"
  [rightVelocity_mPerS] -> Product/2
  Trigonometric Function1/1 -> Product1/3
  Trigonometric Function2/1 -> Product/3
  theta_rad/1 -> Trigonometric Function2/1, Trigonometric Function1/1

== system AreaCoverageTestHarness/Robot/OrientationCalculator/Localization/ThetaCalc ==
  W_radPerS : Inport
  thetaOld : Inport  Port=2
  OrientationCalc : Subsystem
  thetaClip : Subsystem
  ThetaClip_rad : Outport
  wires:
  thetaClip/1(ThetaClip_rad) -> ThetaClip_rad/1
  W_radPerS/1 -> OrientationCalc/1(W_radPerS)
  OrientationCalc/1(Theta_rad) -> thetaClip/1(Theta_rad)
  thetaOld/1 -> OrientationCalc/2(theta_OLD)

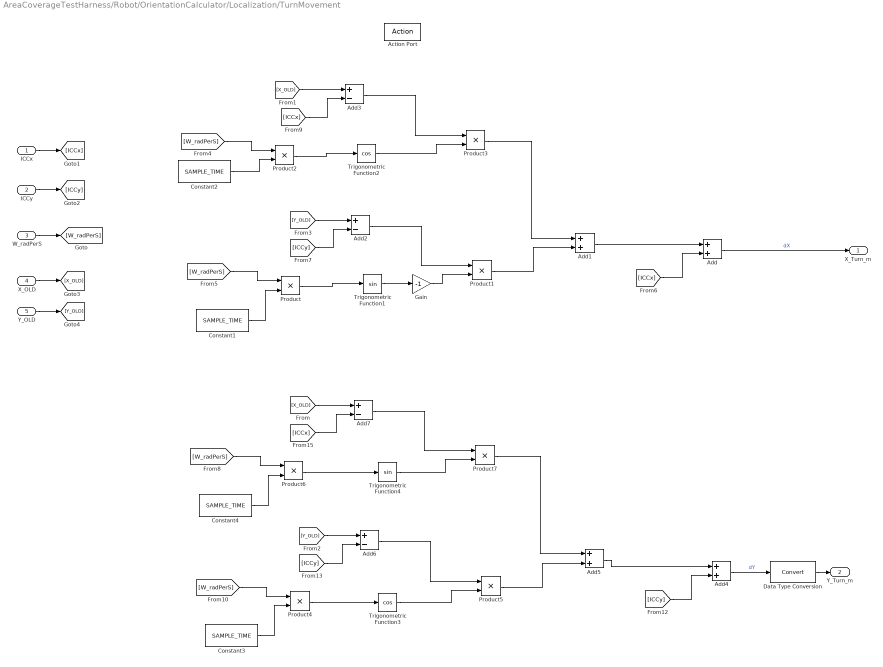
== system AreaCoverageTestHarness/Robot/OrientationCalculator/Localization/TurnMovement ==
  ICCx : Inport
  ICCy : Inport  Port=2
  W_radPerS : Inport  Port=3
  X_OLD : Inport  Port=4
  Y_OLD : Inport  Port=5
  Action Port : ActionPort  ActionType=then
      settings: AttributesFormatString=%<InitializeStates>
  Add{,1,4..5} (4 alike) : Sum
  Add{2..3,6..7} (4 alike) : Sum  Inputs=+-
  Constant{1..4} (4 alike) : Constant  Value=SAMPLE_TIME  SampleTime=-1
  Data Type Conversion : DataTypeConversion
  Gain : Gain  Gain=-1
  Product{,1..7} (8 alike) : Product
  Trigonometric Function1 : Trigonometry
  Trigonometric Function2 : Trigonometry  Operator=cos
  Trigonometric Function3 : Trigonometry  Operator=cos
  Trigonometric Function4 : Trigonometry
  X_Turn_m : Outport  InitialOutput=initXSim
      settings: AttributesFormatString=|
      | %<InitialOutput>
      | %<OutputWhenDisabled>
  Y_Turn_m : Outport  Port=2  InitialOutput=initYSim
      settings: AttributesFormatString=|
      | %<InitialOutput>
      | %<OutputWhenDisabled>
  wires:
  [W_radPerS] -> Product/1
  Gain/1 -> Product1/2
  [ICCx] -> Add/2
  Add2/1 -> Product1/1
  Add1/1 -> Add/1
  Product1/1 -> Add1/2
  Constant1/1 -> Product/2
  Add3/1 -> Product3/1
  Add/1 -> X_Turn_m/1  "dX"
  Trigonometric Function1/1 -> Gain/1
  [ICCy] -> Add2/2
  Constant2/1 -> Product2/2
  Trigonometric Function2/1 -> Product3/2
  [ICCx] -> Add3/2
  [W_radPerS] -> Product2/1
  Product3/1 -> Add1/1
  Add6/1 -> Product5/1
  [ICCy] -> Add4/2
  Product5/1 -> Add5/2
  Product7/1 -> Add5/1
  Add7/1 -> Product7/1
  Trigonometric Function3/1 -> Product5/2
  Add5/1 -> Add4/1
  Trigonometric Function4/1 -> Product7/2
  [W_radPerS] -> Product4/1
  Add4/1 -> Data Type Conversion/1  "dY"
  [ICCy] -> Add6/2
  [ICCx] -> Add7/2
  Constant3/1 -> Product4/2
  [W_radPerS] -> Product6/1
  Constant4/1 -> Product6/2
  W_radPerS/1 -> [W_radPerS]
  ICCx/1 -> [ICCx]
  ICCy/1 -> [ICCy]
  X_OLD/1 -> [X_OLD]
  [X_OLD] -> Add7/1
  [X_OLD] -> Add3/1
  Y_OLD/1 -> [Y_OLD]
  [Y_OLD] -> Add6/1
  [Y_OLD] -> Add2/1
  Product/1 -> Trigonometric Function1/1
  Product2/1 -> Trigonometric Function2/1
  Product6/1 -> Trigonometric Function4/1
  Product4/1 -> Trigonometric Function3/1
  Data Type Conversion/1 -> Y_Turn_m/1

== system AreaCoverageTestHarness/Robot/OrientationCalculator/Localization/thetaFilter ==
  thetaRaw : Inport
  Add : Sum  Inputs=+-
  Add1 : Sum
  Constant : Constant  Value=360
  Constant1 : Constant  Value=360
  Constant2 : Constant  Value=0
  Relational Operator : RelationalOperator  Operator=>  OutDataTypeStr=boolean  RndMeth=Nearest
  Relational Operator1 : RelationalOperator  Operator=<  OutDataTypeStr=boolean  RndMeth=Nearest
  Switch : Switch  Criteria=u2 > Threshold
  Switch1 : Switch  Criteria=u2 > Threshold
  thetaFiltered : Outport
  wires:
  thetaRaw/1 -> Switch1/3, Add/1, Add1/2, Relational Operator1/1, Relational Operator/1
  Constant/1 -> Add1/1, Relational Operator/2
  Relational Operator/1 -> Switch/2
  Constant1/1 -> Add/2
  Add/1 -> Switch/1
  Constant2/1 -> Relational Operator1/2
  Relational Operator1/1 -> Switch1/2
  Add1/1 -> Switch1/1
  Switch1/1 -> Switch/3
  Switch/1 -> thetaFiltered/1

== system AreaCoverageTestHarness/Robot/OrientationCalculator/VelocityCalculator/LeftPhysicalMotorModel ==
  pos : Inport
  neg : Inport  Port=2
  LoadTorq : Inport  Port=3
  PhysicalMotorModel_Call : Inport  Port=4
  PulseGenerator : Subsystem  TreatAsAtomicUnit=on  SystemSampleTime=0.0001
  Rate Transition : RateTransition
  Terminator : Terminator
  Terminator1 : Terminator
  motorModel : Subsystem
  Ia_A : Outport  OutputWhenDisabled=reset  InitialOutput=0
  pulseGenerator : Outport  Port=2  InitialOutput=0
  Velocity_mmPerS : Outport  Port=3  OutputWhenDisabled=reset  InitialOutput=0
  physDistDebug_mm : Outport  Port=4
  wires:
  PulseGenerator/1(pulseGenerator) -> pulseGenerator/1
  pos/1 -> motorModel/1(pos)
  neg/1 -> motorModel/2(neg)
  LoadTorq/1 -> motorModel/3(LoadTorq)
  PhysicalMotorModel_Call/1 -> motorModel/Trigger
  PulseGenerator/2(physDistDebug_mm) -> physDistDebug_mm/1
  motorModel/2(omega_radPerS) -> Rate Transition/1
  Rate Transition/1 -> PulseGenerator/1(omega_radPerS)
  motorModel/4(DIRECT) -> Terminator/1
  motorModel/3(theta_rad) -> Terminator1/1
  motorModel/5(Velocity_mmPerS) -> Velocity_mmPerS/1
  motorModel/1(Ia_A) -> Ia_A/1

== system AreaCoverageTestHarness/Robot/OrientationCalculator/VelocityCalculator/RightPhysicalMotorModel ==
  pos : Inport
  neg : Inport  Port=2
  LoadTorq : Inport  Port=3
  PhysicalMotorModel_Call : Inport  Port=4
  PulseGenerator : Subsystem  TreatAsAtomicUnit=on  SystemSampleTime=0.0001
  Rate Transition : RateTransition
  Terminator : Terminator
  Terminator1 : Terminator
  motorModel : Subsystem
  Ia_A : Outport  OutputWhenDisabled=reset  InitialOutput=0
  pulseGenerator : Outport  Port=2  InitialOutput=0
  Velocity_mmPerS : Outport  Port=3  OutputWhenDisabled=reset  InitialOutput=0
  physDistDebug_mm : Outport  Port=4
  wires:
  PulseGenerator/2(physDistDebug_mm) -> physDistDebug_mm/1
  PhysicalMotorModel_Call/1 -> motorModel/Trigger
  motorModel/2(omega_radPerS) -> Rate Transition/1
  motorModel/1(Ia_A) -> Ia_A/1
  LoadTorq/1 -> motorModel/3(LoadTorq)
  neg/1 -> motorModel/2(neg)
  pos/1 -> motorModel/1(pos)
  PulseGenerator/1(pulseGenerator) -> pulseGenerator/1
  Rate Transition/1 -> PulseGenerator/1(omega_radPerS)
  motorModel/5(Velocity_mmPerS) -> Velocity_mmPerS/1
  motorModel/4(DIRECT) -> Terminator/1
  motorModel/3(theta_rad) -> Terminator1/1

== system AreaCoverageTestHarness/Robot/OrientationCalculator/Localization/R_Calc/If Action Subsystem1 ==
  rightVelocity_mPerS : Inport
  leftVelocity_mPerS : Inport  Port=2
  Action Port : ActionPort  InitializeStates=reset  ActionType=then
      settings: AttributesFormatString=%<InitializeStates>
  Add : Sum
  Add1 : Sum  Inputs=+-
  Constant3 : Constant  Value=ROB_LENG_m
  Constant4 : Constant  Value=2
  Divide1 : Product  Inputs=*/
  Divide2 : Product  Inputs=*/
  Product1 : Product
  R : Outport  OutputWhenDisabled=reset  InitialOutput=999999999999
      settings: AttributesFormatString=|
      | Mode: %<OutputWhenDisabled>
      | InitialOuput: %<InitialOutput>
  wires:
  rightVelocity_mPerS/1 -> Add1/1, Add/1
  Add1/1 -> Divide2/2
  Add/1 -> Divide2/1
  Divide1/1 -> Product1/2
  Divide2/1 -> Product1/1
  Constant3/1 -> Divide1/1
  Product1/1 -> R/1
  leftVelocity_mPerS/1 -> Add1/2, Add/2
  Constant4/1 -> Divide1/2

== system AreaCoverageTestHarness/Robot/OrientationCalculator/Localization/ThetaCalc/OrientationCalc ==
  W_radPerS : Inport
  theta_OLD : Inport  Port=2
  Add : Sum
  Constant4 : Constant  Value=SAMPLE_TIME  SampleTime=-1
  Product : Product
  Theta_rad : Outport
  wires:
  theta_OLD/1 -> Add/2
  Constant4/1 -> Product/2
  W_radPerS/1 -> Product/1
  Add/1 -> Theta_rad/1
  Product/1 -> Add/1

== system AreaCoverageTestHarness/Robot/OrientationCalculator/Localization/ThetaCalc/thetaClip ==
  Theta_rad : Inport
  Add : Sum  Inputs=+-
  Add1 : Sum
  Constant1 : Constant  Value=2*pi
  Constant2 : Constant  Value=0
  Constant3 : Constant  Value=2*pi
  Relational Operator : RelationalOperator  Operator=>  OutDataTypeStr=boolean  RndMeth=Nearest
  Relational Operator1 : RelationalOperator  Operator=<  OutDataTypeStr=boolean  RndMeth=Nearest
  Switch : Switch  Criteria=u2 ~= 0
  Switch1 : Switch  Criteria=u2 ~= 0
  ThetaClip_rad : Outport
  wires:
  Theta_rad/1 -> Switch1/3, Add/1, Add1/2, Relational Operator1/1, Relational Operator/1
  Constant3/1 -> Add1/1, Relational Operator/2
  Relational Operator/1 -> Switch/2
  Constant1/1 -> Add/2
  Add/1 -> Switch/1
  Constant2/1 -> Relational Operator1/2
  Relational Operator1/1 -> Switch1/2
  Add1/1 -> Switch1/1
  Switch1/1 -> Switch/3
  Switch/1 -> ThetaClip_rad/1

== system AreaCoverageTestHarness/Robot/OrientationCalculator/VelocityCalculator/LeftPhysicalMotorModel/PulseGenerator ==
  note: Justification: Cannot implement encoder with interrupt due to limitation in arduino UNO....
      | two digital pins as interrupt d2 and d3. encoder input is from value 0 to 190 adc value,
      | which most probably will not be able to fire the interrupt.
  note: TODO: Relate CAL_mm_Per_Ticks to pulse generator so it produces the same as reality.
  omega_radPerS : Inport
  Abs : Abs
  Chart2 : Stateflow chart  TreatAsAtomicUnit=on
  Data Type Conversion : DataTypeConversion  OutDataTypeStr=single
  Discrete-Time Integrator : DiscreteIntegrator  SampleTime=-1  ICPrevOutput=DiscIntNeverNeededParam  ICPrevScaledInput=DiscIntNeverNeededParam
  Gain : Gain  Gain=halfWheel_mm
  pulseGenerator : Outport
  physDistDebug_mm : Outport  Port=2
  wires:
  Data Type Conversion/1 -> physDistDebug_mm/1
  Discrete-Time Integrator/1 -> Abs/1, Gain/1  "theta_rad"
  Gain/1 -> Data Type Conversion/1
  Abs/1 -> Chart2/1(currentTheta)
  omega_radPerS/1 -> Discrete-Time Integrator/1
  Chart2/1(pulseFlg) -> pulseGenerator/1
